simulink model "truesystem"  (R2020a)
settings: Solver=VariableStepAuto  StartTime=0.0  StopTime=stoptimetotal  RelTol=1e-3
values from neighbouring files (symbols this model uses):
  battery = load('params/battery.mat').battery    [prognostics.m]    (also in workspace_1.mat = )
  IC = load('params/IC_HoverAt10ftOcto.mat').IC    [prognostics.m]    (also in workspace_1.mat = )
  Motor1 = load('params/Motors/Motor1.mat').Motor    [prognostics.m]    (also in workspace_1.mat = )
  Motor2 = load('params/Motors/Motor2.mat').Motor    [prognostics.m]    (also in workspace_1.mat = )
  Motor3 = load('params/Motors/Motor3.mat').Motor    [prognostics.m]    (also in workspace_1.mat = )
  Motor4 = load('params/Motors/Motor4.mat').Motor    [prognostics.m]    (also in workspace_1.mat = )
  Motor5 = load('params/Motors/Motor5.mat').Motor    [prognostics.m]    (also in workspace_1.mat = )
  Motor6 = load('params/Motors/Motor6.mat').Motor    [prognostics.m]    (also in workspace_1.mat = )
  Motor7 = load('params/Motors/Motor7.mat').Motor    [prognostics.m]    (also in workspace_1.mat = )
  Motor8 = load('params/Motors/Motor8.mat').Motor    [prognostics.m]    (also in workspace_1.mat = )
  octomodel = load('params/octoModel.mat').octomodel    [prognostics.m]    (also in workspace_1.mat = )
  sampletimetraj = 1    [prognostics.m]    (also in workspace_1.mat)
undefined symbols (not defined in the file or in its folder): DiscIntNeverNeededParam, mu_wind
libraries: dspstat3 x9, sharedTrackingLibrary x4
(part 1 of 2)
settings Model: Creator=Researcher  LastModifiedBy=darrahts
settings DataIOCC: ReturnWorkspaceOutputs=off
settings DebuggingCC: ArithmeticOperatorsInVariantConditions=warning
settings SFSimCC: SimUseLocalCustomCode=off  CustomCodeUndefinedFunction=UseInterfaceOnly
settings RTWCC: RTWUseLocalCustomCode=off

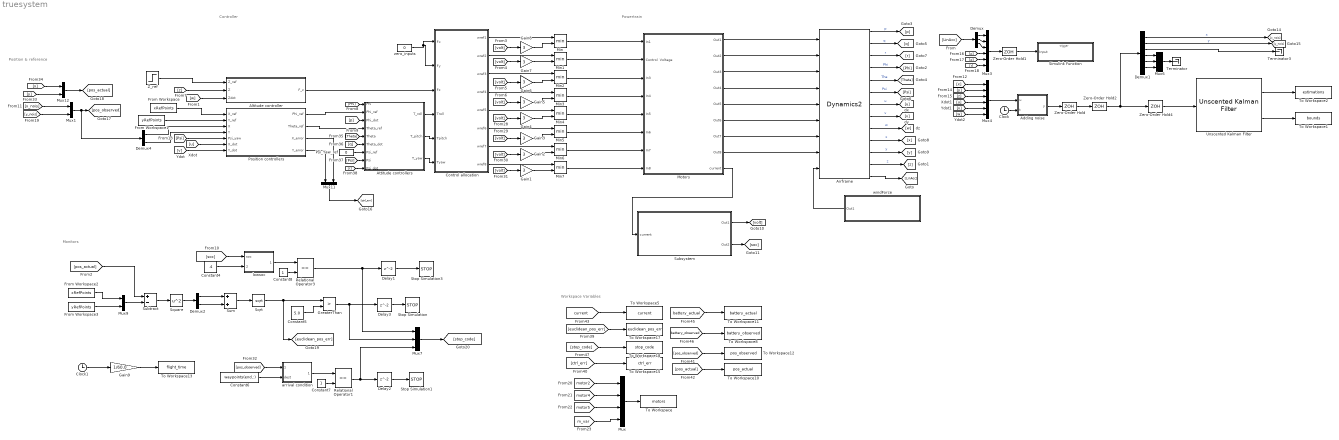
== system truesystem ==
  note: Powertrain
  note: Position & reference
  note: Controller
  note: Monitors
  note: Workspace Variables
  Adding noise : MATLAB Function  TreatAsAtomicUnit=on  SystemSampleTime=octomodel.sampletime
  Airframe : M-S-Function  FunctionName=Dynamics2  Parameters=octomodel, IC
  Altitude controller : Subsystem
  Attitude controllers : Subsystem
  Clock : Clock
  Clock1 : Clock
  Constant4 : Constant  Value=.4
  Constant5 : Constant  Value=5.0
  Constant6 : Constant  Value=waypoints(end,:)
  Constant7 : Constant
  Constant8 : Constant
  Control allocation : MATLAB Function  TreatAsAtomicUnit=on
  Delay1 : Delay
  Delay2 : Delay
  Delay3 : Delay
  Demux : Demux  Outputs=3
  Demux1 : Demux  Outputs=6
  Demux2 : Demux  Outputs=2
  Demux4 : Demux  Outputs=2
  From Workspace : FromWorkspace  VariableName=xRefPoints  SampleTime=sampletimetraj
  From Workspace1 : FromWorkspace  VariableName=yRefPoints  SampleTime=sampletimetraj
  From Workspace2 : FromWorkspace  VariableName=xRefPoints  SampleTime=sampletimetraj
  From Workspace3 : FromWorkspace  VariableName=yRefPoints  SampleTime=sampletimetraj
  Gain{1..8} (8 alike) : Gain  Gain=3
  Gain9 : Gain  Gain=1/60.0
  GreaterThan : RelationalOperator  Operator=>  OutDataTypeStr=boolean  RndMeth=Simplest
  Min{,1..7} (8 alike) : MinMax  Inputs=2
  Motors : Subsystem
  Mux : Mux
  Mux{1,9,11..12} (4 alike) : Mux  Inputs=2
  Mux3 : Mux  Inputs=6
  Mux4 : Mux  Inputs=6
  Mux6 : Mux  Inputs=3
  Mux7 : Mux  Inputs=3
  Position controllers : Subsystem
  Psi_Yaw_ref : Constant  Value=0
  Relational Operator1 : RelationalOperator  Operator===  OutDataTypeStr=boolean  RndMeth=Simplest
  Relational Operator3 : RelationalOperator  Operator===  OutDataTypeStr=boolean  RndMeth=Simplest
  Simulink Function : Subsystem  TreatAsAtomicUnit=on
  Sqrt : Sqrt  SaturateOnIntegerOverflow=on
  Square : Math  Operator=square  SaturateOnIntegerOverflow=on
  Stop Simulation : Stop
  Stop Simulation1 : Stop
  Stop Simulation3 : Stop
  Subsystem : Subsystem
  Subtract : Sum  Inputs=+-
  Sum : Sum
  Terminator : Terminator
  Terminator3 : Terminator
  To Workspace : ToWorkspace  VariableName=motors  SaveFormat=Timeseries  SampleTime=-1
  To Workspace1 : ToWorkspace  VariableName=bounds  SaveFormat=Timeseries  SampleTime=battery.dt
  To Workspace10 : ToWorkspace  VariableName=pos_actual  SaveFormat=Timeseries  SampleTime=-1
  To Workspace11 : ToWorkspace  VariableName=battery_actual  SaveFormat=Timeseries  SampleTime=-1
  To Workspace12 : ToWorkspace  VariableName=pos_observed  SaveFormat=Timeseries  SampleTime=-1
  To Workspace13 : ToWorkspace  VariableName=flight_time  SaveFormat=Timeseries  SampleTime=-1
  To Workspace15 : ToWorkspace  VariableName=ctrl_err  SaveFormat=Timeseries  SampleTime=-1
  To Workspace17 : ToWorkspace  VariableName=euclidean_pos_err  SaveFormat=Timeseries  SampleTime=-1
  To Workspace18 : ToWorkspace  VariableName=stop_code  SaveFormat=Timeseries  SampleTime=-1
  To Workspace2 : ToWorkspace  VariableName=estimations  SaveFormat=Timeseries  SampleTime=battery.dt
  To Workspace5 : ToWorkspace  VariableName=current  SaveFormat=Timeseries  SampleTime=-1
      settings: Save2DSignal=2-D array (concatenate along first dimension)
  To Workspace8 : ToWorkspace  VariableName=battery_observed  SaveFormat=Timeseries  SampleTime=-1
  Unscented Kalman Filter : sharedTrackingLibrary/Unscented Kalman Filter  StateTransitionFcn=stateTransitionFn  HasAdditiveProcessNoise=Additive  ProcessNoise=PositionEstimator.SigmaW  HasTimeVaryingProcessNoise=off  HasStateTransitionFcnExtraArgument=0  InitialState=IC.state  InitialStateCovariance=PositionEstimator.SigmaX  Alpha=0.75  Beta=2  Kappa=0  MeasurementFcn1=positionMeasTransitionFunction  HasMeasurementEnablePort1=off  HasAdditiveMeasurementNoise1=Additive  MeasurementNoise1=PositionEstimator.SigmaV  HasTimeVaryingMeasurementNoise1=off  HasMeasurementFcnExtraArgument1=0  MeasurementFcn2=myMeasurementFcn  HasMeasurementEnablePort2=off  HasAdditiveMeasurementNoise2=Additive  MeasurementNoise2=1  HasTimeVaryingMeasurementNoise2=off  HasMeasurementFcnExtraArgument2=0  MeasurementFcn3=myMeasurementFcn  HasMeasurementEnablePort3=off  HasAdditiveMeasurementNoise3=Additive  MeasurementNoise3=1  HasTimeVaryingMeasurementNoise3=off  HasMeasurementFcnExtraArgument3=0  MeasurementFcn4=myMeasurementFcn  HasMeasurementEnablePort4=off  HasAdditiveMeasurementNoise4=Additive  MeasurementNoise4=1  HasTimeVaryingMeasurementNoise4=off  HasMeasurementFcnExtraArgument4=0  MeasurementFcn5=myMeasurementFcn  HasMeasurementEnablePort5=off  HasAdditiveMeasurementNoise5=Additive  MeasurementNoise5=1  HasTimeVaryingMeasurementNoise5=off  HasMeasurementFcnExtraArgument5=0  EnableMultirate=off  StateTransitionFcnSampleTime=0.01  MeasurementFcn1SampleTime=1  MeasurementFcn2SampleTime=1  MeasurementFcn3SampleTime=1  MeasurementFcn4SampleTime=1  MeasurementFcn5SampleTime=1  UseCurrentEstimator=on  OutputStateCovariance=on  DataType=double  SampleTime=battery.dt  NumberOfMeasurements=1
      settings: SourceProductBaseCode=CT,DR,TF,ID,NV,AR,RO,VE
  Z_ref : Step  Before=3  After=3  SampleTime=0
  Zero-Order Hold : ZeroOrderHold
  Zero-Order Hold1 : ZeroOrderHold  SampleTime=octomodel.sampletime
  Zero-Order Hold2 : ZeroOrderHold  SampleTime=octomodel.sampletime
  Zero-Order Hold4 : ZeroOrderHold  SampleTime=battery.dt
  arrival condition : MATLAB Function  TreatAsAtomicUnit=on
  lowsoc : MATLAB Function  TreatAsAtomicUnit=on
  windForce : Subsystem
  zero_inputs : Constant  Value=0
  wires:
  Airframe/1 -> [p]  "p"
  Airframe/2 -> [q]  "q"
  Airframe/3 -> [r]  "r"
  Airframe/4 -> [Phi]  "Phi"
  Airframe/5 -> [Theta]  "The"
  Airframe/6 -> [Psi]  "Psi"
  Airframe/11 -> [y]  "y"
  Airframe/12 -> [z]  "z"
  Airframe/7 -> [u]  "u"
  Airframe/10 -> [x]  "x"
  Airframe/9 -> [w]  "w"
  Airframe/8 -> [v]  "v"
  Motors/3(Out3) -> Airframe/3
  Motors/1(Out1) -> Airframe/1
  Motors/8(Out8) -> Airframe/8
  Motors/7(Out7) -> Airframe/7
  Motors/6(Out6) -> Airframe/6
  Motors/5(Out5) -> Airframe/5
  Motors/4(Out4) -> Airframe/4
  Motors/2(Out2) -> Airframe/2
  Airframe/13 -> [LinAcc]
  [LinAcc] -> Demux/1
  Demux/1 -> Mux3/1
  Demux/2 -> Mux3/2
  Demux/3 -> Mux3/3
  [p] -> Mux3/4
  [q] -> Mux3/5
  [r] -> Mux3/6
  Zero-Order Hold1/1 -> Simulink Function/1(Input)
  Mux3/1 -> Zero-Order Hold1/1
  Clock/1 -> Adding noise/2(t)
  [y] -> Mux4/2
  Zero-Order Hold2/1 -> Zero-Order Hold4/1, Demux1/1
  Adding noise/1(y) -> Zero-Order Hold/1
  Unscented Kalman Filter/1 -> To Workspace2/1
  [x] -> Mux4/1
  [w] -> Mux4/6
  [z] -> Mux4/3
  [v] -> Mux4/5
  [u] -> Mux4/4
  Mux4/1 -> Adding noise/1(u)
  Unscented Kalman Filter/2 -> To Workspace1/1
  Zero-Order Hold/1 -> Zero-Order Hold2/1
  Demux1/3 -> Terminator3/1
  Mux6/1 -> Terminator/1
  Demux1/5 -> Mux6/2
  Demux1/4 -> Mux6/1
  Demux1/6 -> Mux6/3
  Demux1/2 -> [y_nois]  "y"
  Demux1/1 -> [x_nois]  "x"
  Zero-Order Hold4/1 -> Unscented Kalman Filter/1
  Control allocation/6(wref6) -> Min5/1
  [volt] -> Gain8/1
  Gain4/1 -> Min4/2
  Attitude controllers/1(T_roll) -> Control allocation/4(Troll)
  Min3/1 -> Motors/4(In4)
  Position controllers/1(Phi_ref) -> Attitude controllers/2(Phi_ref)
  [r] -> Attitude controllers/9(Psi_dot)
  Z_ref/1 -> Altitude controller/1(Z_ref)
  Gain5/1 -> Min3/2
  Gain1/1 -> Min7/2
  Attitude controllers/3(T_yaw) -> Control allocation/6(Tyaw)
  Control allocation/8(wref8) -> Min7/1
  Mux11/1 -> [ctrl_err]
  [x] -> Mux12/1
  Min7/1 -> Motors/8(In8)
  [Psi] -> Position controllers/5(Psi_yaw)
  [w] -> Altitude controller/3(Zdot)
  [u] -> Position controllers/6(X_dot)
  Demux4/1 -> Position controllers/3(X)
  From Workspace/1 -> Position controllers/1(X_ref)
  Control allocation/7(wref7) -> Min6/1
  Demux4/2 -> Position controllers/4(Y)
  Position controllers/3(X_error) -> Mux11/2
  Min2/1 -> Motors/3(In3)
  Control allocation/3(wref3) -> Min2/1
  [volt] -> Gain2/1
  Min4/1 -> Motors/5(In5)
  Attitude controllers/2(T_pitch) -> Control allocation/5(Tpitch)
  [Theta] -> Attitude controllers/5(Theta)
  Position controllers/2(Theta_ref) -> Attitude controllers/4(Theta_ref)
  Control allocation/1(wref1) -> Min/1
  Altitude controller/1(F_z) -> Control allocation/3(Fz)
  [y] -> Mux12/2
  [Phi] -> Attitude controllers/1(Phi)
  [z] -> Altitude controller/2(Z)
  [volt] -> Gain5/1
  Position controllers/4(Y_error) -> Mux11/1
  Gain2/1 -> Min6/2
  Min5/1 -> Motors/6(In6)
  Control allocation/4(wref4) -> Min3/1
  Min1/1 -> Motors/2(Control  Voltage)
  [volt] -> Gain4/1
  Control allocation/5(wref5) -> Min4/1
  [volt] -> Gain3/1
  Control allocation/2(wref2) -> Min1/1
  From Workspace1/1 -> Position controllers/2(Y_ref)
  [v] -> Position controllers/7(Y_dot)
  [Psi] -> Attitude controllers/8(Psi)
  [volt] -> Gain1/1
  Min6/1 -> Motors/7(In7)
  [volt] -> Gain7/1
  zero_inputs/1 -> Control allocation/1(Fx), Control allocation/2(Fy)
  Min/1 -> Motors/1(In1)
  Gain8/1 -> Min/2
  [q] -> Attitude controllers/6(Theta_dot)
  Psi_Yaw_ref/1 -> Attitude controllers/7(Psi_ref)
  [p] -> Attitude controllers/3(Phi_dot)
  [volt] -> Gain6/1
  Gain3/1 -> Min5/2
  Gain7/1 -> Min1/2
  Mux12/1 -> [pos_actual]
  Gain6/1 -> Min2/2
  Constant7/1 -> Relational Operator1/2
  Mux7/1 -> [stop_code]
  lowsoc/1(lowsoc) -> Relational Operator3/1
  Constant6/1 -> arrival condition/2(dest)
  Demux2/2 -> Sum/2
  Delay2/1 -> Stop Simulation1/1
  Constant5/1 -> GreaterThan/2
  Gain9/1 -> To Workspace13/1
  arrival condition/1(arrived) -> Relational Operator1/1
  Demux2/1 -> Sum/1
  [pos_actual] -> Subtract/1
  Mux9/1 -> Subtract/2
  Delay1/1 -> Stop Simulation3/1
  From Workspace3/1 -> Mux9/2
  Constant4/1 -> lowsoc/2(threshold)
  Clock1/1 -> Gain9/1
  Sum/1 -> Sqrt/1
  [soc] -> lowsoc/1(soc)
  GreaterThan/1 -> Mux7/2, Delay3/1
  Sqrt/1 -> [euclidean_pos_err], GreaterThan/1
  Square/1 -> Demux2/1
  Subtract/1 -> Square/1
  From Workspace2/1 -> Mux9/1
  Constant8/1 -> Relational Operator3/2
  [pos_observed] -> arrival condition/1(currentpos)
  Relational Operator1/1 -> Mux7/3, Delay2/1
  Delay3/1 -> Stop Simulation/1
  Relational Operator3/1 -> Mux7/1, Delay1/1
  [stop_code] -> To Workspace18/1
  [pos_actual] -> To Workspace10/1
  [pos_observed] -> To Workspace12/1
  [ctrl_err] -> To Workspace15/1
  [battery_actual] -> To Workspace11/1
  [current] -> To Workspace5/1
  [battery_observed] -> To Workspace8/1
  [euclidean_pos_err] -> To Workspace17/1
  Motors/9(current) -> Subsystem/1(current)
  Subsystem/1(Out1) -> [volt]
  Subsystem/2(Out2) -> [soc]
  Mux1/1 -> Demux4/1, [pos_observed]
  [x_nois] -> Mux1/1
  [y_nois] -> Mux1/2
  windForce/1(Out1) -> Airframe/9
  [motor2] -> Mux/1
  [m_var] -> Mux/4
  [motor5] -> Mux/3
  [motor4] -> Mux/2
  Mux/1 -> To Workspace/1

== system truesystem/Altitude controller ==
  Z_ref : Inport
  Z : Inport  Port=2
  Zdot : Inport  Port=3
  Add : Sum  Inputs=+++
  Add2 : Sum  Inputs=+-
  Constant2 : Constant  Value=octomodel.g*octomodel.mass
  Kdz : Gain  Gain=-3
  Kpz : Gain  Gain=-10
  mass : Gain  Gain=octomodel.mass
  mass1 : Gain  Gain=octomodel.mass
  F_z : Outport  VectorParamsAs1DForOutWhenUnconnected=off
  wires:
  Add2/1 -> Kpz/1
  Constant2/1 -> Add/1
  Z/1 -> Add2/1
  Add/1 -> F_z/1
  Z_ref/1 -> Add2/2
  Zdot/1 -> Kdz/1
  Kpz/1 -> mass/1
  Kdz/1 -> mass1/1
  mass1/1 -> Add/3
  mass/1 -> Add/2

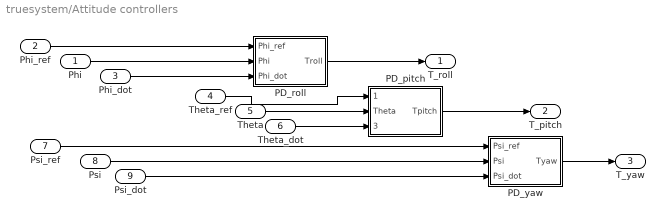
== system truesystem/Attitude controllers ==
  Phi : Inport
  Phi_ref : Inport  Port=2
  Phi_dot : Inport  Port=3
  Theta_ref : Inport  Port=4
  Theta : Inport  Port=5
  Theta_dot : Inport  Port=6
  Psi_ref : Inport  Port=7
  Psi : Inport  Port=8
  Psi_dot : Inport  Port=9
  PD_pitch : Subsystem
  PD_roll : Subsystem
  PD_yaw : Subsystem
  T_roll : Outport  VectorParamsAs1DForOutWhenUnconnected=off
  T_pitch : Outport  Port=2  VectorParamsAs1DForOutWhenUnconnected=off
  T_yaw : Outport  Port=3  VectorParamsAs1DForOutWhenUnconnected=off
  wires:
  PD_yaw/1(Tyaw) -> T_yaw/1
  PD_roll/1(Troll) -> T_roll/1
  Theta_ref/1 -> PD_pitch/1(Theta_ref)
  Theta_dot/1 -> PD_pitch/3(Theta_dot)
  PD_pitch/1(Tpitch) -> T_pitch/1
  Phi/1 -> PD_roll/2(Phi)
  Psi_dot/1 -> PD_yaw/3(Psi_dot)
  Psi_ref/1 -> PD_yaw/1(Psi_ref)
  Theta/1 -> PD_pitch/2(Theta)
  Phi_dot/1 -> PD_roll/3(Phi_dot)
  Psi/1 -> PD_yaw/2(Psi)
  Phi_ref/1 -> PD_roll/1(Phi_ref)

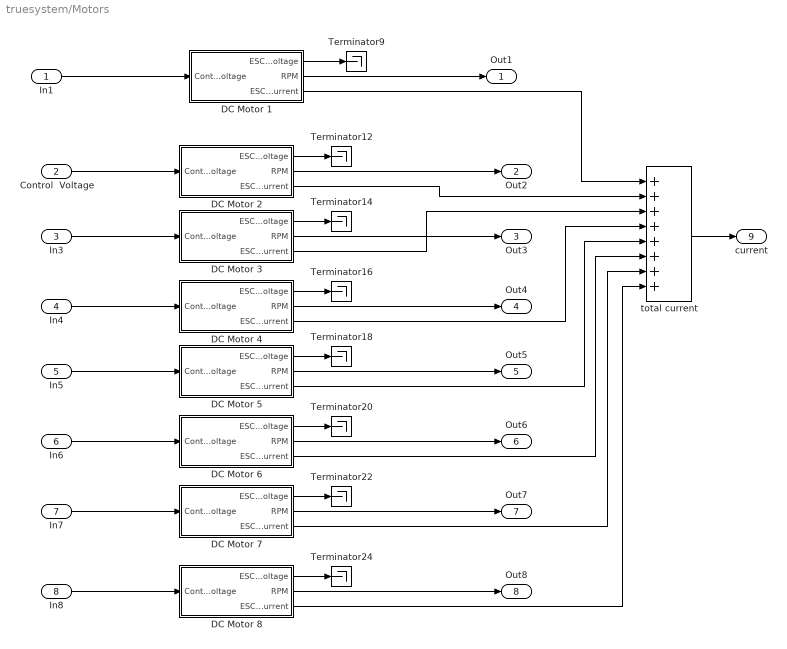
== system truesystem/Motors ==
  In1 : Inport
  Control  Voltage : Inport  Port=2
  In3 : Inport  Port=3
  In4 : Inport  Port=4
  In5 : Inport  Port=5
  In6 : Inport  Port=6
  In7 : Inport  Port=7
  In8 : Inport  Port=8
  "DC Motor 1 " : Subsystem
  DC Motor 2 : Subsystem
  DC Motor 3 : Subsystem
  DC Motor 4 : Subsystem
  DC Motor 5 : Subsystem
  DC Motor 6 : Subsystem
  DC Motor 7 : Subsystem
  DC Motor 8 : Subsystem
  Terminator{9,12,14,16,18,20,22,24} (8 alike) : Terminator
  total current : Sum  Inputs=++++++++
  Out1 : Outport  VectorParamsAs1DForOutWhenUnconnected=off
  Out2 : Outport  Port=2  VectorParamsAs1DForOutWhenUnconnected=off
  Out3 : Outport  Port=3  VectorParamsAs1DForOutWhenUnconnected=off
  Out4 : Outport  Port=4  VectorParamsAs1DForOutWhenUnconnected=off
  Out5 : Outport  Port=5  VectorParamsAs1DForOutWhenUnconnected=off
  Out6 : Outport  Port=6  VectorParamsAs1DForOutWhenUnconnected=off
  Out7 : Outport  Port=7  VectorParamsAs1DForOutWhenUnconnected=off
  Out8 : Outport  Port=8  VectorParamsAs1DForOutWhenUnconnected=off
  current : Outport  Port=9  VectorParamsAs1DForOutWhenUnconnected=off
  wires:
  DC Motor 5/1(ESC Voltage) -> Terminator18/1
  DC Motor 6/3(ESC Current) -> total current/6
  DC Motor 7/3(ESC Current) -> total current/7
  DC Motor 7/1(ESC Voltage) -> Terminator22/1
  DC Motor 6/1(ESC Voltage) -> Terminator20/1
  DC Motor 5/3(ESC Current) -> total current/5
  DC Motor 8/3(ESC Current) -> total current/8
  "DC Motor 1 "/3(ESC Current) -> total current/1
  "DC Motor 1 "/1(ESC Voltage) -> Terminator9/1
  DC Motor 2/3(ESC Current) -> total current/2
  DC Motor 2/1(ESC Voltage) -> Terminator12/1
  DC Motor 3/1(ESC Voltage) -> Terminator14/1
  DC Motor 4/3(ESC Current) -> total current/4
  DC Motor 3/3(ESC Current) -> total current/3
  DC Motor 5/2(RPM) -> Out5/1
  DC Motor 4/1(ESC Voltage) -> Terminator16/1
  DC Motor 8/1(ESC Voltage) -> Terminator24/1
  DC Motor 7/2(RPM) -> Out7/1
  DC Motor 2/2(RPM) -> Out2/1
  DC Motor 3/2(RPM) -> Out3/1
  DC Motor 4/2(RPM) -> Out4/1
  DC Motor 6/2(RPM) -> Out6/1
  DC Motor 8/2(RPM) -> Out8/1
  "DC Motor 1 "/2(RPM) -> Out1/1
  In1/1 -> "DC Motor 1 "/1(Control  Voltage)
  In7/1 -> DC Motor 7/1(Control  Voltage)
  In8/1 -> DC Motor 8/1(Control  Voltage)
  In6/1 -> DC Motor 6/1(Control  Voltage)
  In5/1 -> DC Motor 5/1(Control  Voltage)
  In4/1 -> DC Motor 4/1(Control  Voltage)
  In3/1 -> DC Motor 3/1(Control  Voltage)
  Control  Voltage/1 -> DC Motor 2/1(Control  Voltage)
  total current/1 -> current/1

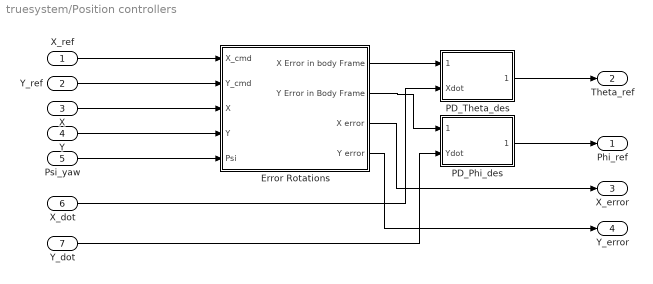
== system truesystem/Position controllers ==
  X_ref : Inport
  Y_ref : Inport  Port=2
  X : Inport  Port=3
  Y : Inport  Port=4
  Psi_yaw : Inport  Port=5
  X_dot : Inport  Port=6
  Y_dot : Inport  Port=7
  Error Rotations : Subsystem
  PD_Phi_des : Subsystem
  PD_Theta_des : Subsystem
  Phi_ref : Outport  VectorParamsAs1DForOutWhenUnconnected=off
  Theta_ref : Outport  Port=2  VectorParamsAs1DForOutWhenUnconnected=off
  X_error : Outport  Port=3  VectorParamsAs1DForOutWhenUnconnected=off
  Y_error : Outport  Port=4  VectorParamsAs1DForOutWhenUnconnected=off
  wires:
  Y/1 -> Error Rotations/4(Y)
  Y_ref/1 -> Error Rotations/2(Y_cmd)
  Error Rotations/4("Y error ") -> Y_error/1
  Error Rotations/3(X error) -> X_error/1
  Error Rotations/1(X Error in body Frame) -> PD_Theta_des/1(Xdot_ref)
  X/1 -> Error Rotations/3(X)
  Y_dot/1 -> PD_Phi_des/2(Ydot)
  PD_Phi_des/1(Phi_des) -> Phi_ref/1
  Error Rotations/2(Y Error in Body Frame) -> PD_Phi_des/1(Ydot_ref)
  Psi_yaw/1 -> Error Rotations/5(Psi)
  PD_Theta_des/1(Theta_des) -> Theta_ref/1
  X_dot/1 -> PD_Theta_des/2(Xdot)
  X_ref/1 -> Error Rotations/1(X_cmd)

== system truesystem/Simulink Function ==
  Input : Inport  PortDimensions=6
  stateTransitionFn : TriggerPort  TriggerType=function-call  IsSimulinkFunction=on  FunctionName=stateTransitionFn  VariantControl=(inherit)
  MATLAB Function : MATLAB Function  TreatAsAtomicUnit=on
  x : ArgIn  DisableCoverage=on  PortDimensions=9  ArgumentName=x
  xNext : ArgOut  DisableCoverage=on  PortDimensions=9  ArgumentName=xNext
  wires:
  x/1 -> MATLAB Function/1("x ")
  MATLAB Function/1(x) -> xNext/1
  Input/1 -> MATLAB Function/2(u)

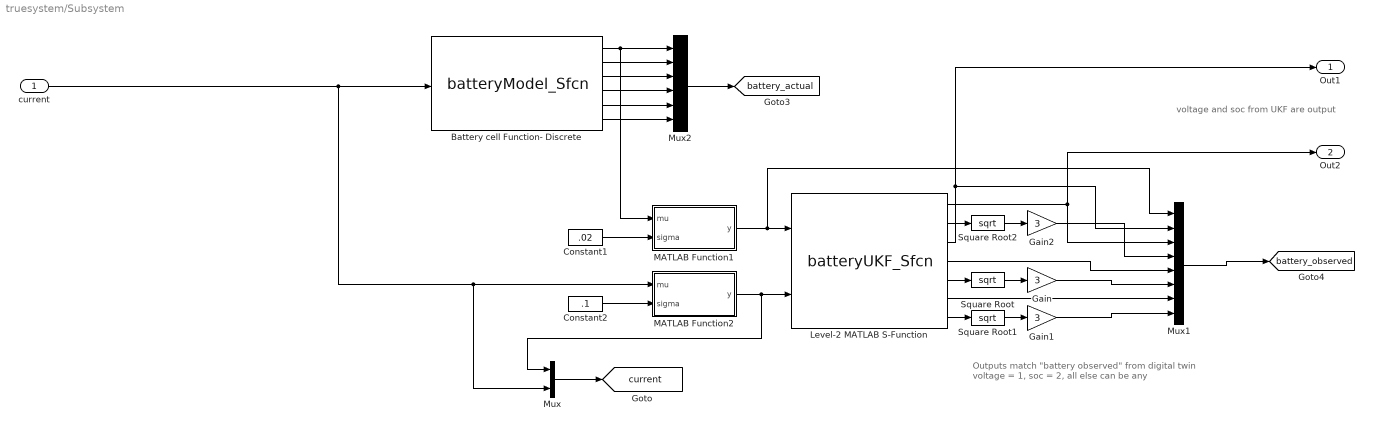
== system truesystem/Subsystem ==
  note: voltage and soc from UKF are output
  note: Outputs match "battery observed" from digital twin
      | voltage = 1, soc = 2, all else can be any
  current : Inport
  Battery cell Function- Discrete : M-S-Function  FunctionName=batteryModel_Sfcn  Parameters=battery, battery.dt
      mask Display:
      | port_label('input', 1, 'current');
      | port_label('output', 1, 'voltage');
      | port_label('output', 2, 'soc');
      | port_label('output', 3, 'R0');
      | port_label('output', 4, 'Ir');
      | port_label('output', 5, 'h');
      | port_label('output', 6, 'Q');
      | 
      | disp("Battery Cell");
  Constant1 : Constant  Value=.02
  Constant2 : Constant  Value=.1
  Gain : Gain  Gain=3
  Gain1 : Gain  Gain=3
  Gain2 : Gain  Gain=3
  Level-2 MATLAB S-Function : M-S-Function  FunctionName=batteryUKF_Sfcn  Parameters=battery, battery.dt, ukfBatteryParams
      mask Display:
      | port_label('input', 1, 'voltage');
      | port_label('input', 2, 'current');
      | port_label('output', 1, 'soc_hat');
      | port_label('output', 2, 'soc_bound');
      | port_label('output', 3, 'voltage_hat');
      | port_label('output', 4, 'r0_hat');
      | port_label('output', 5, 'r0_bound');
      | port_label('output', 6, 'q_hat');
      | port_label('output', 7, 'q_bound');
      | 
      | disp("UKF");
  MATLAB Function1 : MATLAB Function  TreatAsAtomicUnit=on
  MATLAB Function2 : MATLAB Function  TreatAsAtomicUnit=on
  Mux : Mux  Inputs=2
  Mux1 : Mux  Inputs=8
  Mux2 : Mux  Inputs=6
  Square Root : Sqrt  SaturateOnIntegerOverflow=on
  Square Root1 : Sqrt  SaturateOnIntegerOverflow=on
  Square Root2 : Sqrt  SaturateOnIntegerOverflow=on
  Out1 : Outport
  Out2 : Outport  Port=2
  tag scope: battery_actual=global, battery_observed=global, current=global
  wires:
  MATLAB Function1/1(y) -> Mux1/1, Level-2 MATLAB S-Function/1
  Constant1/1 -> MATLAB Function1/2(sigma)
  Level-2 MATLAB S-Function/5 -> Square Root/1
  Square Root/1 -> Gain/1
  Battery cell Function- Discrete/6 -> Mux2/6
  Battery cell Function- Discrete/1 -> MATLAB Function1/1(mu), Mux2/1
  Battery cell Function- Discrete/5 -> Mux2/5
  Battery cell Function- Discrete/2 -> Mux2/2
  Battery cell Function- Discrete/4 -> Mux2/4
  Mux2/1 -> [battery_actual]
  Battery cell Function- Discrete/3 -> Mux2/3
  Square Root1/1 -> Gain1/1
  Square Root2/1 -> Gain2/1
  Level-2 MATLAB S-Function/2 -> Square Root2/1
  Level-2 MATLAB S-Function/7 -> Square Root1/1
  Level-2 MATLAB S-Function/3 -> Mux1/2, Out1/1
  Level-2 MATLAB S-Function/1 -> Out2/1, Mux1/3
  Gain2/1 -> Mux1/4
  Level-2 MATLAB S-Function/4 -> Mux1/5
  Gain/1 -> Mux1/6
  Level-2 MATLAB S-Function/6 -> Mux1/7
  Gain1/1 -> Mux1/8
  Mux1/1 -> [battery_observed]
  Constant2/1 -> MATLAB Function2/2(sigma)
  current/1 -> Mux/2, MATLAB Function2/1(mu), Battery cell Function- Discrete/1
  MATLAB Function2/1(y) -> Mux/1, Level-2 MATLAB S-Function/2
  Mux/1 -> [current]

== system truesystem/windForce ==
  Constant10 : Constant  Value=[0;0;0]
  Gain : Gain  Gain=.5
  Manual Switch1 : ManualSwitch  CurrentSetting=0
  Mux9 : Mux  Inputs=3
  Random Number : RandomNumber  Mean=mu_wind  Variance=.5  Seed=37
  Random Number1 : RandomNumber  Mean=mu_wind  Variance=.5  Seed=41
  Random Number2 : RandomNumber  Mean=mu_wind  Variance=.5
  Out1 : Outport
  wires:
  Random Number1/1 -> Mux9/2
  Mux9/1 -> Gain/1
  Manual Switch1/1 -> Out1/1
  Random Number2/1 -> Mux9/3
  Random Number/1 -> Mux9/1
  Constant10/1 -> Manual Switch1/1
  Gain/1 -> Manual Switch1/2

== system truesystem/Attitude controllers/PD_pitch ==
  Theta_ref : Inport
  Theta : Inport  Port=2
  Theta_dot : Inport  Port=3
  Add : Sum  Inputs=-+
  Gain : Gain  Gain=3
  Gain1 : Gain
  Gain2 : Gain  Gain=-1
  Sum : Sum  Inputs=|++
  Tpitch : Outport  VectorParamsAs1DForOutWhenUnconnected=off
  wires:
  Gain2/1 -> Tpitch/1
  Gain/1 -> Sum/1
  Theta/1 -> Add/2
  Add/1 -> Gain/1
  Gain1/1 -> Sum/2
  Sum/1 -> Gain2/1
  Theta_dot/1 -> Gain1/1
  Theta_ref/1 -> Add/1

== system truesystem/Attitude controllers/PD_roll ==
  Phi_ref : Inport
  Phi : Inport  Port=2
  Phi_dot : Inport  Port=3
  Add : Sum  Inputs=-+
  Gain : Gain  Gain=3
  Gain1 : Gain
  Gain2 : Gain  Gain=-1
  Sum : Sum  Inputs=|++
  Troll : Outport  VectorParamsAs1DForOutWhenUnconnected=off
  wires:
  Phi_ref/1 -> Add/1
  Phi_dot/1 -> Gain1/1
  Sum/1 -> Gain2/1
  Gain1/1 -> Sum/2
  Add/1 -> Gain/1
  Phi/1 -> Add/2
  Gain/1 -> Sum/1
  Gain2/1 -> Troll/1

== system truesystem/Attitude controllers/PD_yaw ==
  Psi_ref : Inport
  Psi : Inport  Port=2
  Psi_dot : Inport  Port=3
  Add : Sum  Inputs=-+
  Gain : Gain  Gain=3
  Gain1 : Gain
  Gain2 : Gain  Gain=-1
  Sum : Sum  Inputs=|++
  Tyaw : Outport  VectorParamsAs1DForOutWhenUnconnected=off
  wires:
  Psi_ref/1 -> Add/1
  Psi_dot/1 -> Gain1/1
  Sum/1 -> Gain2/1
  Gain1/1 -> Sum/2
  Add/1 -> Gain/1
  Psi/1 -> Add/2
  Gain/1 -> Sum/1
  Gain2/1 -> Tyaw/1

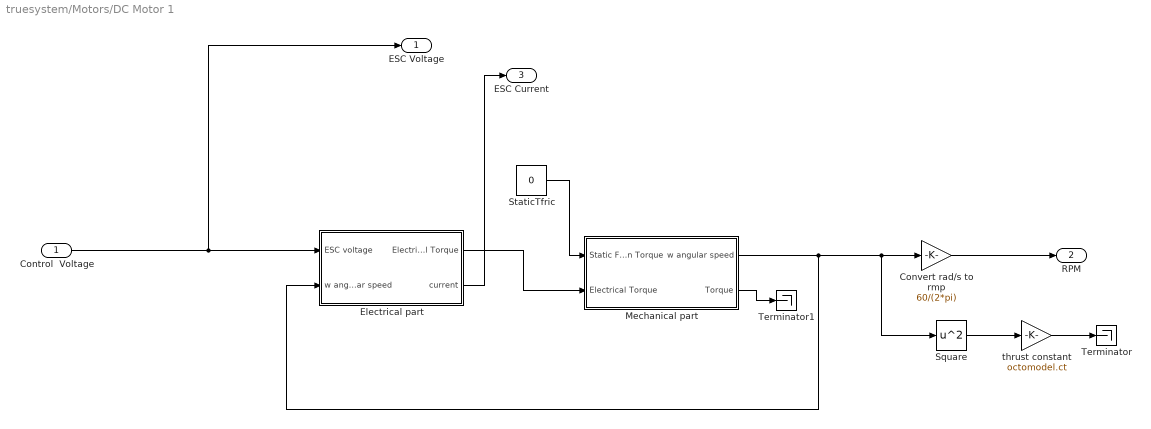
== system truesystem/Motors/DC Motor 1  ==
  Control  Voltage : Inport
  Convert rad/s to rmp : Gain  Gain=60/(2*pi)
  Electrical part : Subsystem
  Mechanical part : Subsystem
  Square : Math  Operator=square  SaturateOnIntegerOverflow=on
  StaticTfric : Constant  Value=0
  Terminator : Terminator
  Terminator1 : Terminator
  thrust constant : Gain  Gain=octomodel.ct
  ESC Voltage : Outport  VectorParamsAs1DForOutWhenUnconnected=off
  RPM : Outport  Port=2  VectorParamsAs1DForOutWhenUnconnected=off
  ESC Current : Outport  Port=3  VectorParamsAs1DForOutWhenUnconnected=off
  wires:
  Electrical part/1(Electrical Torque) -> Mechanical part/2(Electrical Torque)
  StaticTfric/1 -> Mechanical part/1(Static Friction Torque)
  Convert rad/s to rmp/1 -> RPM/1
  Square/1 -> thrust constant/1
  thrust constant/1 -> Terminator/1
  Mechanical part/2(Torque) -> Terminator1/1
  Electrical part/2(current) -> ESC Current/1
  Control  Voltage/1 -> ESC Voltage/1, Electrical part/1(ESC voltage)
  Mechanical part/1(w angular speed) -> Electrical part/2(w angular speed), Square/1, Convert rad/s to rmp/1

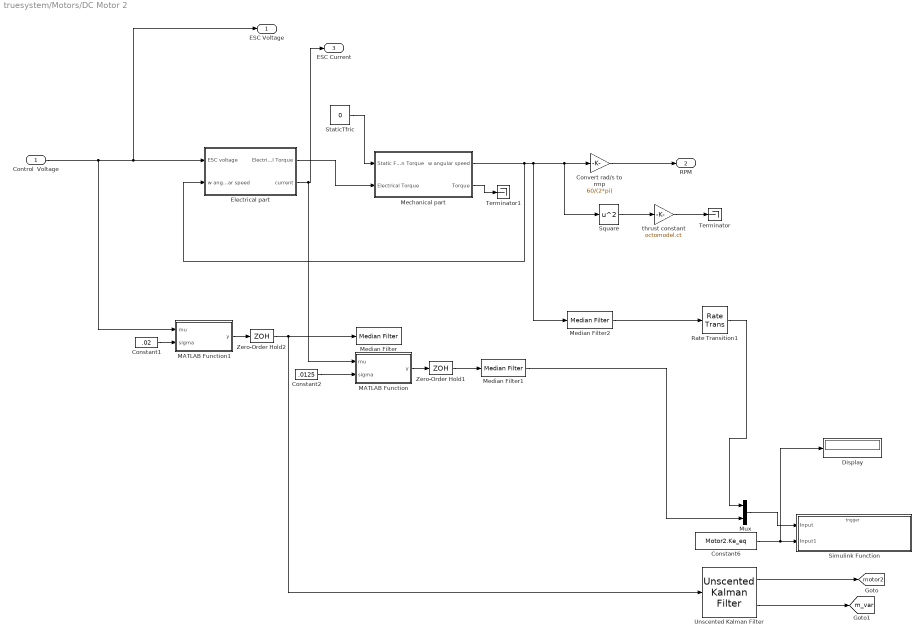
== system truesystem/Motors/DC Motor 2 ==
  Control  Voltage : Inport
  Constant1 : Constant  Value=.02
  Constant2 : Constant  Value=.0125
  Constant6 : Constant  Value=Motor2.Ke_eq
  Convert rad/s to rmp : Gain  Gain=60/(2*pi)
  Display : Display
  Electrical part : Subsystem
  MATLAB Function : MATLAB Function  TreatAsAtomicUnit=on
  MATLAB Function1 : MATLAB Function  TreatAsAtomicUnit=on
  Mechanical part : Subsystem
  Median Filter : dspstat3/Median Filter  WindowLength=5  SimulateUsing=Interpreted execution
      settings: SourceProductBaseCode=DS
  Median Filter1 : dspstat3/Median Filter  WindowLength=5  SimulateUsing=Interpreted execution
      settings: SourceProductBaseCode=DS
  Median Filter2 : dspstat3/Median Filter  WindowLength=5  SimulateUsing=Interpreted execution
      settings: SourceProductBaseCode=DS
  Mux : Mux  Inputs=2
  Rate Transition1 : RateTransition  OutPortSampleTime=octomodel.sampletime
  Simulink Function : Subsystem  TreatAsAtomicUnit=on
  Square : Math  Operator=square  SaturateOnIntegerOverflow=on
  StaticTfric : Constant  Value=0
  Terminator : Terminator
  Terminator1 : Terminator
  Unscented Kalman Filter : sharedTrackingLibrary/Unscented Kalman Filter  StateTransitionFcn=MotorTransitionFcn  HasAdditiveProcessNoise=Additive  ProcessNoise=0.001  HasTimeVaryingProcessNoise=off  HasStateTransitionFcnExtraArgument=0  InitialState=MotorEstimator.Rinit  InitialStateCovariance=0.001  Alpha=0.0001  Beta=2  Kappa=0  MeasurementFcn1=MotorMeasurementFcn2  HasMeasurementEnablePort1=off  HasAdditiveMeasurementNoise1=Additive  MeasurementNoise1=0.02  HasTimeVaryingMeasurementNoise1=off  HasMeasurementFcnExtraArgument1=0  MeasurementFcn2=myMeasurementFcn  HasMeasurementEnablePort2=off  HasAdditiveMeasurementNoise2=Additive  MeasurementNoise2=1  HasTimeVaryingMeasurementNoise2=off  HasMeasurementFcnExtraArgument2=0  MeasurementFcn3=myMeasurementFcn  HasMeasurementEnablePort3=off  HasAdditiveMeasurementNoise3=Additive  MeasurementNoise3=1  HasTimeVaryingMeasurementNoise3=off  HasMeasurementFcnExtraArgument3=0  MeasurementFcn4=myMeasurementFcn  HasMeasurementEnablePort4=off  HasAdditiveMeasurementNoise4=Additive  MeasurementNoise4=1  HasTimeVaryingMeasurementNoise4=off  HasMeasurementFcnExtraArgument4=0  MeasurementFcn5=myMeasurementFcn  HasMeasurementEnablePort5=off  HasAdditiveMeasurementNoise5=Additive  MeasurementNoise5=1  HasTimeVaryingMeasurementNoise5=off  HasMeasurementFcnExtraArgument5=0  EnableMultirate=off  StateTransitionFcnSampleTime=1  MeasurementFcn1SampleTime=1  MeasurementFcn2SampleTime=1  MeasurementFcn3SampleTime=1  MeasurementFcn4SampleTime=1  MeasurementFcn5SampleTime=1  UseCurrentEstimator=on  OutputStateCovariance=on  DataType=double  SampleTime=octomodel.sampletime  NumberOfMeasurements=1
      settings: SourceProductBaseCode=CT,DR,TF,ID,NV,AR,RO,VE
  Zero-Order Hold1 : ZeroOrderHold  SampleTime=octomodel.sampletime
  Zero-Order Hold2 : ZeroOrderHold  SampleTime=octomodel.sampletime
  thrust constant : Gain  Gain=octomodel.ct
  ESC Voltage : Outport  VectorParamsAs1DForOutWhenUnconnected=off
  RPM : Outport  Port=2  VectorParamsAs1DForOutWhenUnconnected=off
  ESC Current : Outport  Port=3  VectorParamsAs1DForOutWhenUnconnected=off
  tag scope: m_var=global, motor2=global
  wires:
  Square/1 -> thrust constant/1
  thrust constant/1 -> Terminator/1
  Convert rad/s to rmp/1 -> RPM/1
  StaticTfric/1 -> Mechanical part/1(Static Friction Torque)
  Electrical part/1(Electrical Torque) -> Mechanical part/2(Electrical Torque)
  Mechanical part/2(Torque) -> Terminator1/1
  Control  Voltage/1 -> MATLAB Function1/1(mu), Electrical part/1(ESC voltage), ESC Voltage/1
  Zero-Order Hold1/1 -> Median Filter1/1
  Mechanical part/1(w angular speed) -> Median Filter2/1, Convert rad/s to rmp/1, Square/1, Electrical part/2(w angular speed)
  Electrical part/2(current) -> MATLAB Function/1(mu), ESC Current/1
  MATLAB Function/1(y) -> Zero-Order Hold1/1
  Constant2/1 -> MATLAB Function/2(sigma)
  Constant1/1 -> MATLAB Function1/2(sigma)
  MATLAB Function1/1(y) -> Zero-Order Hold2/1
  Median Filter2/1 -> Rate Transition1/1
  Median Filter1/1 -> Mux/2
  Mux/1 -> Simulink Function/1(Input)
  Rate Transition1/1 -> Mux/1
  Unscented Kalman Filter/1 -> [motor2]
  Constant6/1 -> Display/1, Simulink Function/2(Input1)
  Zero-Order Hold2/1 -> Unscented Kalman Filter/1, Median Filter/1
  Unscented Kalman Filter/2 -> [m_var]

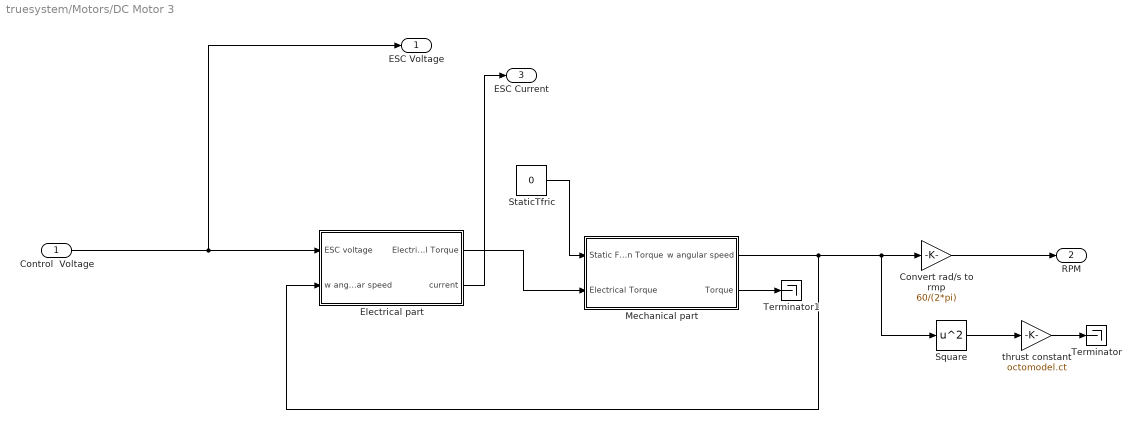
== system truesystem/Motors/DC Motor 3 ==
  Control  Voltage : Inport
  Convert rad/s to rmp : Gain  Gain=60/(2*pi)
  Electrical part : Subsystem
  Mechanical part : Subsystem
  Square : Math  Operator=square  SaturateOnIntegerOverflow=on
  StaticTfric : Constant  Value=0
  Terminator : Terminator
  Terminator1 : Terminator
  thrust constant : Gain  Gain=octomodel.ct
  ESC Voltage : Outport  VectorParamsAs1DForOutWhenUnconnected=off
  RPM : Outport  Port=2  VectorParamsAs1DForOutWhenUnconnected=off
  ESC Current : Outport  Port=3  VectorParamsAs1DForOutWhenUnconnected=off
  wires:
  Electrical part/1(Electrical Torque) -> Mechanical part/2(Electrical Torque)
  StaticTfric/1 -> Mechanical part/1(Static Friction Torque)
  Control  Voltage/1 -> ESC Voltage/1, Electrical part/1(ESC voltage)
  Electrical part/2(current) -> ESC Current/1
  Convert rad/s to rmp/1 -> RPM/1
  Mechanical part/1(w angular speed) -> Electrical part/2(w angular speed), Square/1, Convert rad/s to rmp/1
  thrust constant/1 -> Terminator/1
  Square/1 -> thrust constant/1
  Mechanical part/2(Torque) -> Terminator1/1

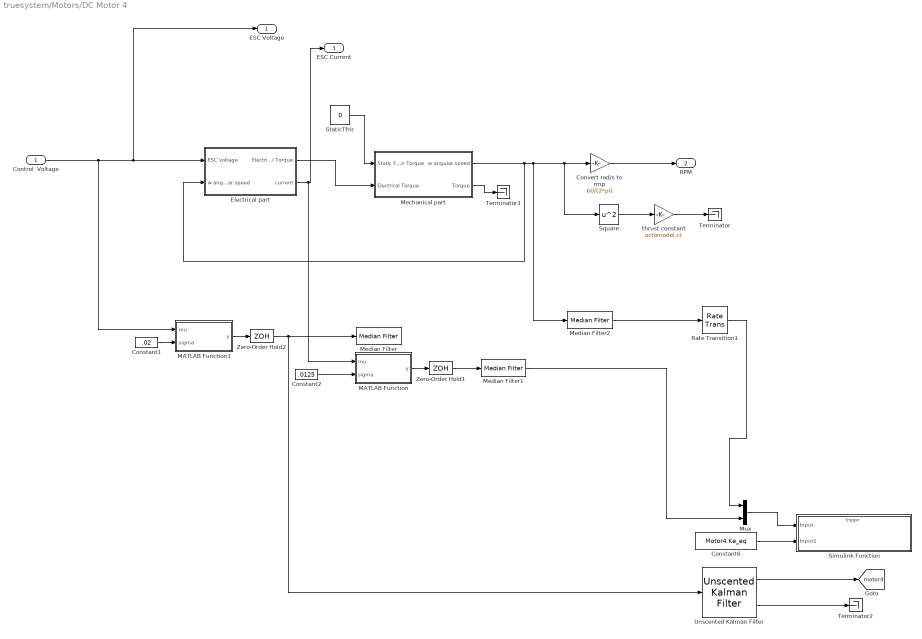
== system truesystem/Motors/DC Motor 4 ==
  Control  Voltage : Inport
  Constant1 : Constant  Value=.02
  Constant2 : Constant  Value=.0125
  Constant6 : Constant  Value=Motor4.Ke_eq
  Convert rad/s to rmp : Gain  Gain=60/(2*pi)
  Electrical part : Subsystem
  MATLAB Function : MATLAB Function  TreatAsAtomicUnit=on
  MATLAB Function1 : MATLAB Function  TreatAsAtomicUnit=on
  Mechanical part : Subsystem
  Median Filter : dspstat3/Median Filter  WindowLength=5  SimulateUsing=Interpreted execution
      settings: SourceProductBaseCode=DS
  Median Filter1 : dspstat3/Median Filter  WindowLength=5  SimulateUsing=Interpreted execution
      settings: SourceProductBaseCode=DS
  Median Filter2 : dspstat3/Median Filter  WindowLength=5  SimulateUsing=Interpreted execution
      settings: SourceProductBaseCode=DS
  Mux : Mux  Inputs=2
  Rate Transition1 : RateTransition  OutPortSampleTime=octomodel.sampletime
  Simulink Function : Subsystem  TreatAsAtomicUnit=on
  Square : Math  Operator=square  SaturateOnIntegerOverflow=on
  StaticTfric : Constant  Value=0
  Terminator : Terminator
  Terminator1 : Terminator
  Terminator2 : Terminator
  Unscented Kalman Filter : sharedTrackingLibrary/Unscented Kalman Filter  StateTransitionFcn=MotorTransitionFcn  HasAdditiveProcessNoise=Additive  ProcessNoise=0.001  HasTimeVaryingProcessNoise=off  HasStateTransitionFcnExtraArgument=0  InitialState=MotorEstimator.Rinit  InitialStateCovariance=0.001  Alpha=0.0001  Beta=2  Kappa=0  MeasurementFcn1=MotorMeasurementFcn4  HasMeasurementEnablePort1=off  HasAdditiveMeasurementNoise1=Additive  MeasurementNoise1=0.02  HasTimeVaryingMeasurementNoise1=off  HasMeasurementFcnExtraArgument1=0  MeasurementFcn2=myMeasurementFcn  HasMeasurementEnablePort2=off  HasAdditiveMeasurementNoise2=Additive  MeasurementNoise2=1  HasTimeVaryingMeasurementNoise2=off  HasMeasurementFcnExtraArgument2=0  MeasurementFcn3=myMeasurementFcn  HasMeasurementEnablePort3=off  HasAdditiveMeasurementNoise3=Additive  MeasurementNoise3=1  HasTimeVaryingMeasurementNoise3=off  HasMeasurementFcnExtraArgument3=0  MeasurementFcn4=myMeasurementFcn  HasMeasurementEnablePort4=off  HasAdditiveMeasurementNoise4=Additive  MeasurementNoise4=1  HasTimeVaryingMeasurementNoise4=off  HasMeasurementFcnExtraArgument4=0  MeasurementFcn5=myMeasurementFcn  HasMeasurementEnablePort5=off  HasAdditiveMeasurementNoise5=Additive  MeasurementNoise5=1  HasTimeVaryingMeasurementNoise5=off  HasMeasurementFcnExtraArgument5=0  EnableMultirate=off  StateTransitionFcnSampleTime=1  MeasurementFcn1SampleTime=1  MeasurementFcn2SampleTime=1  MeasurementFcn3SampleTime=1  MeasurementFcn4SampleTime=1  MeasurementFcn5SampleTime=1  UseCurrentEstimator=on  OutputStateCovariance=on  DataType=double  SampleTime=octomodel.sampletime  NumberOfMeasurements=1
      settings: SourceProductBaseCode=CT,DR,TF,ID,NV,AR,RO,VE
  Zero-Order Hold1 : ZeroOrderHold  SampleTime=octomodel.sampletime
  Zero-Order Hold2 : ZeroOrderHold  SampleTime=octomodel.sampletime
  thrust constant : Gain  Gain=octomodel.ct
  ESC Voltage : Outport  VectorParamsAs1DForOutWhenUnconnected=off
  RPM : Outport  Port=2  VectorParamsAs1DForOutWhenUnconnected=off
  ESC Current : Outport  Port=3  VectorParamsAs1DForOutWhenUnconnected=off
  tag scope: motor4=global
  wires:
  Square/1 -> thrust constant/1
  thrust constant/1 -> Terminator/1
  Convert rad/s to rmp/1 -> RPM/1
  StaticTfric/1 -> Mechanical part/1(Static Friction Torque)
  Electrical part/1(Electrical Torque) -> Mechanical part/2(Electrical Torque)
  Mechanical part/2(Torque) -> Terminator1/1
  Control  Voltage/1 -> MATLAB Function1/1(mu), Electrical part/1(ESC voltage), ESC Voltage/1
  Zero-Order Hold1/1 -> Median Filter1/1
  Mechanical part/1(w angular speed) -> Median Filter2/1, Convert rad/s to rmp/1, Square/1, Electrical part/2(w angular speed)
  Electrical part/2(current) -> MATLAB Function/1(mu), ESC Current/1
  MATLAB Function/1(y) -> Zero-Order Hold1/1
  Constant2/1 -> MATLAB Function/2(sigma)
  Constant1/1 -> MATLAB Function1/2(sigma)
  MATLAB Function1/1(y) -> Zero-Order Hold2/1
  Median Filter2/1 -> Rate Transition1/1
  Median Filter1/1 -> Mux/2
  Mux/1 -> Simulink Function/1(Input)
  Rate Transition1/1 -> Mux/1
  Unscented Kalman Filter/1 -> [motor4]
  Constant6/1 -> Simulink Function/2(Input1)
  Zero-Order Hold2/1 -> Unscented Kalman Filter/1, Median Filter/1
  Unscented Kalman Filter/2 -> Terminator2/1

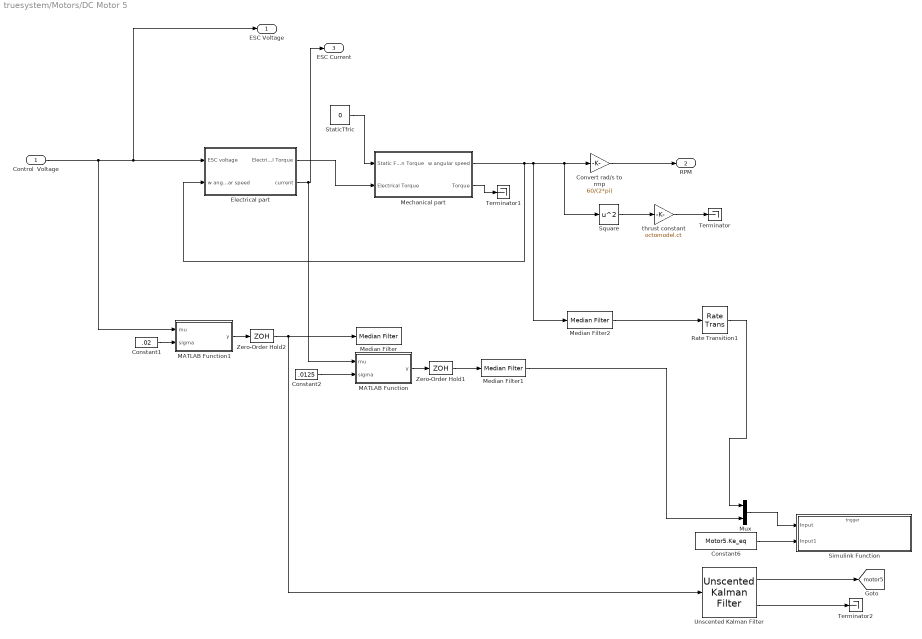
== system truesystem/Motors/DC Motor 5 ==
  Control  Voltage : Inport
  Constant1 : Constant  Value=.02
  Constant2 : Constant  Value=.0125
  Constant6 : Constant  Value=Motor5.Ke_eq
  Convert rad/s to rmp : Gain  Gain=60/(2*pi)
  Electrical part : Subsystem
  MATLAB Function : MATLAB Function  TreatAsAtomicUnit=on
  MATLAB Function1 : MATLAB Function  TreatAsAtomicUnit=on
  Mechanical part : Subsystem
  Median Filter : dspstat3/Median Filter  WindowLength=5  SimulateUsing=Interpreted execution
      settings: SourceProductBaseCode=DS
  Median Filter1 : dspstat3/Median Filter  WindowLength=5  SimulateUsing=Interpreted execution
      settings: SourceProductBaseCode=DS
  Median Filter2 : dspstat3/Median Filter  WindowLength=5  SimulateUsing=Interpreted execution
      settings: SourceProductBaseCode=DS
  Mux : Mux  Inputs=2
  Rate Transition1 : RateTransition  OutPortSampleTime=octomodel.sampletime
  Simulink Function : Subsystem  TreatAsAtomicUnit=on
  Square : Math  Operator=square  SaturateOnIntegerOverflow=on
  StaticTfric : Constant  Value=0
  Terminator : Terminator
  Terminator1 : Terminator
  Terminator2 : Terminator
  Unscented Kalman Filter : sharedTrackingLibrary/Unscented Kalman Filter  StateTransitionFcn=MotorTransitionFcn  HasAdditiveProcessNoise=Additive  ProcessNoise=0.001  HasTimeVaryingProcessNoise=off  HasStateTransitionFcnExtraArgument=0  InitialState=MotorEstimator.Rinit  InitialStateCovariance=0.001  Alpha=0.0001  Beta=2  Kappa=0  MeasurementFcn1=MotorMeasurementFcn5  HasMeasurementEnablePort1=off  HasAdditiveMeasurementNoise1=Additive  MeasurementNoise1=0.02  HasTimeVaryingMeasurementNoise1=off  HasMeasurementFcnExtraArgument1=0  MeasurementFcn2=myMeasurementFcn  HasMeasurementEnablePort2=off  HasAdditiveMeasurementNoise2=Additive  MeasurementNoise2=1  HasTimeVaryingMeasurementNoise2=off  HasMeasurementFcnExtraArgument2=0  MeasurementFcn3=myMeasurementFcn  HasMeasurementEnablePort3=off  HasAdditiveMeasurementNoise3=Additive  MeasurementNoise3=1  HasTimeVaryingMeasurementNoise3=off  HasMeasurementFcnExtraArgument3=0  MeasurementFcn4=myMeasurementFcn  HasMeasurementEnablePort4=off  HasAdditiveMeasurementNoise4=Additive  MeasurementNoise4=1  HasTimeVaryingMeasurementNoise4=off  HasMeasurementFcnExtraArgument4=0  MeasurementFcn5=myMeasurementFcn  HasMeasurementEnablePort5=off  HasAdditiveMeasurementNoise5=Additive  MeasurementNoise5=1  HasTimeVaryingMeasurementNoise5=off  HasMeasurementFcnExtraArgument5=0  EnableMultirate=off  StateTransitionFcnSampleTime=1  MeasurementFcn1SampleTime=1  MeasurementFcn2SampleTime=1  MeasurementFcn3SampleTime=1  MeasurementFcn4SampleTime=1  MeasurementFcn5SampleTime=1  UseCurrentEstimator=on  OutputStateCovariance=on  DataType=double  SampleTime=octomodel.sampletime  NumberOfMeasurements=1
      settings: SourceProductBaseCode=CT,DR,TF,ID,NV,AR,RO,VE
  Zero-Order Hold1 : ZeroOrderHold  SampleTime=octomodel.sampletime
  Zero-Order Hold2 : ZeroOrderHold  SampleTime=octomodel.sampletime
  thrust constant : Gain  Gain=octomodel.ct
  ESC Voltage : Outport  VectorParamsAs1DForOutWhenUnconnected=off
  RPM : Outport  Port=2  VectorParamsAs1DForOutWhenUnconnected=off
  ESC Current : Outport  Port=3  VectorParamsAs1DForOutWhenUnconnected=off
  tag scope: motor5=global
  wires:
  Square/1 -> thrust constant/1
  thrust constant/1 -> Terminator/1
  Convert rad/s to rmp/1 -> RPM/1
  StaticTfric/1 -> Mechanical part/1(Static Friction Torque)
  Electrical part/1(Electrical Torque) -> Mechanical part/2(Electrical Torque)
  Mechanical part/2(Torque) -> Terminator1/1
  Control  Voltage/1 -> MATLAB Function1/1(mu), Electrical part/1(ESC voltage), ESC Voltage/1
  Zero-Order Hold1/1 -> Median Filter1/1
  Mechanical part/1(w angular speed) -> Median Filter2/1, Convert rad/s to rmp/1, Square/1, Electrical part/2(w angular speed)
  Electrical part/2(current) -> MATLAB Function/1(mu), ESC Current/1
  MATLAB Function/1(y) -> Zero-Order Hold1/1
  Constant2/1 -> MATLAB Function/2(sigma)
  Constant1/1 -> MATLAB Function1/2(sigma)
  MATLAB Function1/1(y) -> Zero-Order Hold2/1
  Median Filter2/1 -> Rate Transition1/1
  Median Filter1/1 -> Mux/2
  Mux/1 -> Simulink Function/1(Input)
  Rate Transition1/1 -> Mux/1
  Unscented Kalman Filter/1 -> [motor5]
  Constant6/1 -> Simulink Function/2(Input1)
  Zero-Order Hold2/1 -> Unscented Kalman Filter/1, Median Filter/1
  Unscented Kalman Filter/2 -> Terminator2/1

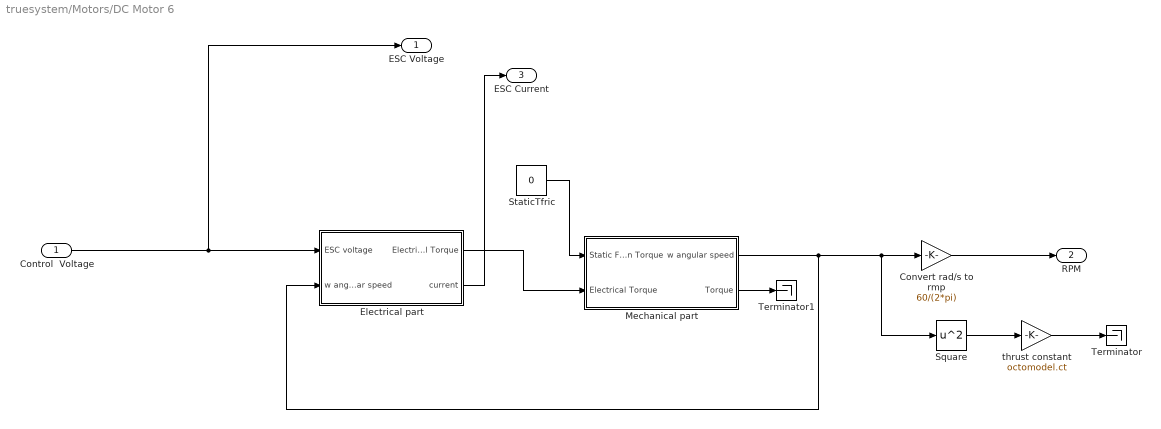
== system truesystem/Motors/DC Motor 6 ==
  Control  Voltage : Inport
  Convert rad/s to rmp : Gain  Gain=60/(2*pi)
  Electrical part : Subsystem
  Mechanical part : Subsystem
  Square : Math  Operator=square  SaturateOnIntegerOverflow=on
  StaticTfric : Constant  Value=0
  Terminator : Terminator
  Terminator1 : Terminator
  thrust constant : Gain  Gain=octomodel.ct
  ESC Voltage : Outport  VectorParamsAs1DForOutWhenUnconnected=off
  RPM : Outport  Port=2  VectorParamsAs1DForOutWhenUnconnected=off
  ESC Current : Outport  Port=3  VectorParamsAs1DForOutWhenUnconnected=off
  wires:
  Square/1 -> thrust constant/1
  Mechanical part/1(w angular speed) -> Convert rad/s to rmp/1, Square/1, Electrical part/2(w angular speed)
  Convert rad/s to rmp/1 -> RPM/1
  Electrical part/2(current) -> ESC Current/1
  Control  Voltage/1 -> Electrical part/1(ESC voltage), ESC Voltage/1
  StaticTfric/1 -> Mechanical part/1(Static Friction Torque)
  Electrical part/1(Electrical Torque) -> Mechanical part/2(Electrical Torque)
  thrust constant/1 -> Terminator/1
  Mechanical part/2(Torque) -> Terminator1/1

== system truesystem/Motors/DC Motor 7 ==
  Control  Voltage : Inport
  Convert rad/s to rmp : Gain  Gain=60/(2*pi)
  Electrical part : Subsystem
  Mechanical part : Subsystem
  Square : Math  Operator=square  SaturateOnIntegerOverflow=on
  StaticTfric : Constant  Value=0
  Terminator : Terminator
  Terminator1 : Terminator
  thrust constant : Gain  Gain=octomodel.ct
  ESC Voltage : Outport  VectorParamsAs1DForOutWhenUnconnected=off
  RPM : Outport  Port=2  VectorParamsAs1DForOutWhenUnconnected=off
  ESC Current : Outport  Port=3  VectorParamsAs1DForOutWhenUnconnected=off
  wires:
  Electrical part/1(Electrical Torque) -> Mechanical part/2(Electrical Torque)
  StaticTfric/1 -> Mechanical part/1(Static Friction Torque)
  Control  Voltage/1 -> ESC Voltage/1, Electrical part/1(ESC voltage)
  Electrical part/2(current) -> ESC Current/1
  Convert rad/s to rmp/1 -> RPM/1
  Mechanical part/1(w angular speed) -> Electrical part/2(w angular speed), Square/1, Convert rad/s to rmp/1
  Square/1 -> thrust constant/1
  thrust constant/1 -> Terminator/1
  Mechanical part/2(Torque) -> Terminator1/1

== system truesystem/Motors/DC Motor 8 ==
  Control  Voltage : Inport
  Convert rad/s to rmp : Gain  Gain=60/(2*pi)
  Electrical part : Subsystem
  Mechanical part : Subsystem
  Square : Math  Operator=square  SaturateOnIntegerOverflow=on
  StaticTfric : Constant  Value=0
  Terminator : Terminator
  Terminator1 : Terminator
  thrust constant : Gain  Gain=octomodel.ct
  ESC Voltage : Outport  VectorParamsAs1DForOutWhenUnconnected=off
  RPM : Outport  Port=2  VectorParamsAs1DForOutWhenUnconnected=off
  ESC Current : Outport  Port=3  VectorParamsAs1DForOutWhenUnconnected=off
  wires:
  Square/1 -> thrust constant/1
  Mechanical part/1(w angular speed) -> Convert rad/s to rmp/1, Square/1, Electrical part/2(w angular speed)
  Convert rad/s to rmp/1 -> RPM/1
  Electrical part/2(current) -> ESC Current/1
  Control  Voltage/1 -> Electrical part/1(ESC voltage), ESC Voltage/1
  StaticTfric/1 -> Mechanical part/1(Static Friction Torque)
  Electrical part/1(Electrical Torque) -> Mechanical part/2(Electrical Torque)
  thrust constant/1 -> Terminator/1
  Mechanical part/2(Torque) -> Terminator1/1

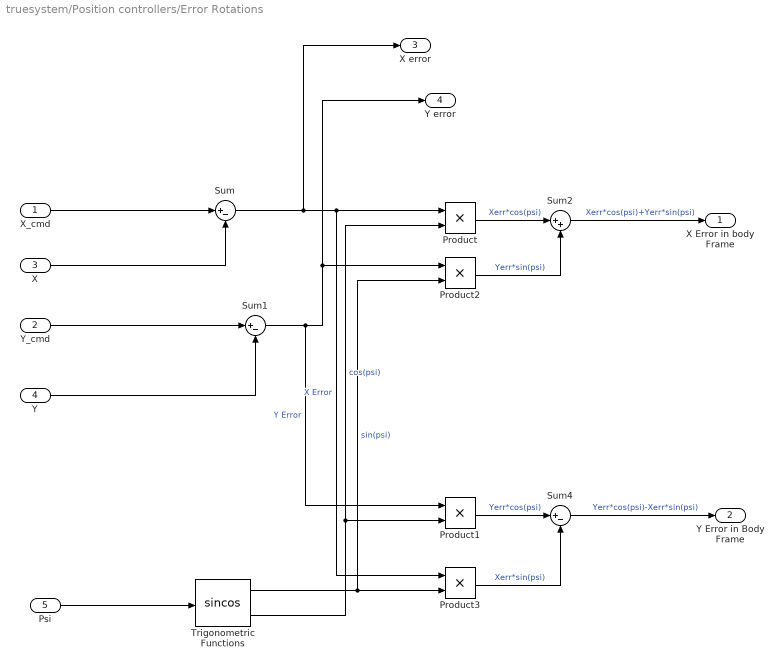
== system truesystem/Position controllers/Error Rotations ==
  X_cmd : Inport
  Y_cmd : Inport  Port=2
  X : Inport  Port=3
  Y : Inport  Port=4
  Psi : Inport  Port=5
  Product{,1..3} (4 alike) : Product
  Sum : Sum  Inputs=|+-
  Sum1 : Sum  Inputs=|+-
  Sum2 : Sum  Inputs=|++
  Sum4 : Sum  Inputs=|+-
  Trigonometric Functions : Trigonometry  Operator=sincos
  X Error in body Frame : Outport  VectorParamsAs1DForOutWhenUnconnected=off
  Y Error in Body Frame : Outport  Port=2  VectorParamsAs1DForOutWhenUnconnected=off
  X error : Outport  Port=3  VectorParamsAs1DForOutWhenUnconnected=off
  "Y error " : Outport  Port=4  VectorParamsAs1DForOutWhenUnconnected=off
  wires:
  Sum4/1 -> Y Error in Body Frame/1  "Yerr*cos(psi)-Xerr*sin(psi)"
  Product3/1 -> Sum4/2  "Xerr*sin(psi)"
  Sum1/1 -> "Y error "/1, Product2/1, Product1/1  "Y Error"
  Trigonometric Functions/1 -> Product2/2, Product3/2  "sin(psi)"
  Sum2/1 -> X Error in body Frame/1  "Xerr*cos(psi)+Yerr*sin(psi)"
  Y_cmd/1 -> Sum1/1
  X_cmd/1 -> Sum/1
  X/1 -> Sum/2
  Y/1 -> Sum1/2
  Sum/1 -> X error/1, Product3/1, Product/1  "X Error"
  Trigonometric Functions/2 -> Product/2, Product1/2  "cos(psi)"
  Product/1 -> Sum2/1  "Xerr*cos(psi)"
  Product2/1 -> Sum2/2  "Yerr*sin(psi)"
  Product1/1 -> Sum4/1  "Yerr*cos(psi)"
  Psi/1 -> Trigonometric Functions/1

== system truesystem/Position controllers/PD_Phi_des ==
  Ydot_ref : Inport
  Ydot : Inport  Port=2
  Add : Sum  Inputs=+-
  Gain : Gain  Gain=0.1
  Gain1 : Gain  Gain=0
  Gain2 : Gain  Gain=-1
  Saturation in radians : Saturate  UpperLimit=12*pi/180  LowerLimit=-12*pi/180
  Sum : Sum  Inputs=|+-
  Phi_des : Outport  VectorParamsAs1DForOutWhenUnconnected=off
  wires:
  Saturation in radians/1 -> Phi_des/1
  Ydot_ref/1 -> Add/1
  Ydot/1 -> Add/2, Gain1/1
  Gain1/1 -> Sum/2
  Add/1 -> Gain/1
  Gain/1 -> Sum/1
  Sum/1 -> Gain2/1
  Gain2/1 -> Saturation in radians/1

== system truesystem/Position controllers/PD_Theta_des ==
  Xdot_ref : Inport
  Xdot : Inport  Port=2
  Add : Sum  Inputs=+-
  Gain : Gain  Gain=0.1
  Gain1 : Gain  Gain=0
  Saturation in radians : Saturate  UpperLimit=12*pi/180  LowerLimit=-12*pi/180
  Sum : Sum  Inputs=|+-
  Theta_des : Outport  VectorParamsAs1DForOutWhenUnconnected=off
  wires:
  Sum/1 -> Saturation in radians/1
  Gain/1 -> Sum/1
  Add/1 -> Gain/1
  Gain1/1 -> Sum/2
  Xdot/1 -> Gain1/1, Add/2
  Xdot_ref/1 -> Add/1
  Saturation in radians/1 -> Theta_des/1

== system truesystem/Motors/DC Motor 1 /Electrical part ==
  ESC voltage : Inport
  w angular speed : Inport  Port=2
  1/R : Gain  Gain=1/Motor1.Req
  Ke (Torque constant)1 : Gain  Gain=Motor1.Ke_eq
  Kt (Torque constant) Kt=Ke for an ideal square wave motor : Gain  Gain=Motor1.Ke_eq
  Saturation : Saturate  UpperLimit=11  LowerLimit=0
  Sum : Sum  Inputs=|+-
  Electrical Torque : Outport  VectorParamsAs1DForOutWhenUnconnected=off
  current : Outport  Port=2  VectorParamsAs1DForOutWhenUnconnected=off
  wires:
  1/R/1 -> Saturation/1  "current i"
  Sum/1 -> 1/R/1
  Kt (Torque constant) Kt=Ke for an ideal square wave motor/1 -> Electrical Torque/1
  Ke (Torque constant)1/1 -> Sum/2
  ESC voltage/1 -> Sum/1
  w angular speed/1 -> Ke (Torque constant)1/1
  Saturation/1 -> Kt (Torque constant) Kt=Ke for an ideal square wave motor/1, current/1

== system truesystem/Motors/DC Motor 1 /Mechanical part ==
  Static Friction Torque : Inport
  Electrical Torque : Inport  Port=2
  1/J Inertia constant : Gain  Gain=1/Motor1.J
  "Df viscous damping coefficient Dynamic Friction coefficient " : Gain  Gain=Motor1.Df
  Discrete-Time Integrator : DiscreteIntegrator  gainval=1  InitialCondition=IC.w1  SampleTime=octomodel.sampletime  ICPrevOutput=DiscIntNeverNeededParam  ICPrevScaledInput=DiscIntNeverNeededParam
  Gain : Gain  Gain=Motor1.cq
  Square : Math  Operator=square  SaturateOnIntegerOverflow=on
  Sum1 : Sum  Inputs=--+-
  w angular speed : Outport  VectorParamsAs1DForOutWhenUnconnected=off
  Torque : Outport  Port=2  VectorParamsAs1DForOutWhenUnconnected=off
  wires:
  1/J Inertia constant/1 -> Discrete-Time Integrator/1
  Static Friction Torque/1 -> Sum1/2
  "Df viscous damping coefficient Dynamic Friction coefficient "/1 -> Sum1/4
  Discrete-Time Integrator/1 -> w angular speed/1, Square/1, "Df viscous damping coefficient Dynamic Friction coefficient "/1  "w angular speed"
  Sum1/1 -> 1/J Inertia constant/1
  Electrical Torque/1 -> Sum1/3
  Gain/1 -> Torque/1, Sum1/1
  Square/1 -> Gain/1

== system truesystem/Motors/DC Motor 2/Electrical part ==
  ESC voltage : Inport
  w angular speed : Inport  Port=2
  1/R : Gain  Gain=1/Motor2.Req
  Ke (Torque constant)1 : Gain  Gain=Motor2.Ke_eq
  Kt (Torque constant) Kt=Ke for an ideal square wave motor : Gain  Gain=Motor2.Ke_eq
  Saturation : Saturate  UpperLimit=11  LowerLimit=0
  Scope1 : Scope
  Scope2 : Scope
  Scope3 : Scope
  Sum : Sum  Inputs=|+-
  Electrical Torque : Outport  VectorParamsAs1DForOutWhenUnconnected=off
  current : Outport  Port=2  VectorParamsAs1DForOutWhenUnconnected=off
  wires:
  Saturation/1 -> current/1, Kt (Torque constant) Kt=Ke for an ideal square wave motor/1, Scope1/1
  w angular speed/1 -> Ke (Torque constant)1/1
  ESC voltage/1 -> Sum/1
  Ke (Torque constant)1/1 -> Sum/2, Scope2/1
  Kt (Torque constant) Kt=Ke for an ideal square wave motor/1 -> Electrical Torque/1
  Sum/1 -> 1/R/1, Scope3/1
  1/R/1 -> Saturation/1  "current i"

== system truesystem/Motors/DC Motor 2/Mechanical part ==
  Static Friction Torque : Inport
  Electrical Torque : Inport  Port=2
  1/J Inertia constant : Gain  Gain=1/Motor2.J
  "Df viscous damping coefficient Dynamic Friction coefficient " : Gain  Gain=Motor2.Df
  Discrete-Time Integrator : DiscreteIntegrator  gainval=1  InitialCondition=IC.w2  SampleTime=octomodel.sampletime  ICPrevOutput=DiscIntNeverNeededParam  ICPrevScaledInput=DiscIntNeverNeededParam
  Gain : Gain  Gain=Motor2.cq
  Square : Math  Operator=square  SaturateOnIntegerOverflow=on
  Sum1 : Sum  Inputs=--+-
  w angular speed : Outport  VectorParamsAs1DForOutWhenUnconnected=off
  Torque : Outport  Port=2  VectorParamsAs1DForOutWhenUnconnected=off
  wires:
  Square/1 -> Gain/1
  Gain/1 -> Sum1/1, Torque/1
  Electrical Torque/1 -> Sum1/3
  Sum1/1 -> 1/J Inertia constant/1
  Discrete-Time Integrator/1 -> "Df viscous damping coefficient Dynamic Friction coefficient "/1, Square/1, w angular speed/1  "w angular speed"
  "Df viscous damping coefficient Dynamic Friction coefficient "/1 -> Sum1/4
  Static Friction Torque/1 -> Sum1/2
  1/J Inertia constant/1 -> Discrete-Time Integrator/1

== system truesystem/Motors/DC Motor 2/Simulink Function ==
  Input : Inport  PortDimensions=2
  Input1 : Inport  Port=2
  MotorMeasurementFcn2 : TriggerPort  TriggerType=function-call  IsSimulinkFunction=on  FunctionName=MotorMeasurementFcn2  VariantControl=(inherit)
  MATLAB Function : MATLAB Function  TreatAsAtomicUnit=on
  x : ArgIn  DisableCoverage=on  ArgumentName=x
  xNext : ArgOut  DisableCoverage=on  ArgumentName=xNext
  wires:
  x/1 -> MATLAB Function/1("x ")
  MATLAB Function/1(x) -> xNext/1
  Input/1 -> MATLAB Function/2(u)
  Input1/1 -> MATLAB Function/3(param)

== system truesystem/Motors/DC Motor 3/Electrical part ==
  ESC voltage : Inport
  w angular speed : Inport  Port=2
  1/R : Gain  Gain=1/Motor3.Req
  Ke (Torque constant)1 : Gain  Gain=Motor3.Ke_eq
  Kt (Torque constant) Kt=Ke for an ideal square wave motor : Gain  Gain=Motor3.Ke_eq
  Saturation : Saturate  UpperLimit=11  LowerLimit=0
  Sum : Sum  Inputs=|+-
  Electrical Torque : Outport  VectorParamsAs1DForOutWhenUnconnected=off
  current : Outport  Port=2  VectorParamsAs1DForOutWhenUnconnected=off
  wires:
  1/R/1 -> Saturation/1  "current i"
  Sum/1 -> 1/R/1
  Kt (Torque constant) Kt=Ke for an ideal square wave motor/1 -> Electrical Torque/1
  Ke (Torque constant)1/1 -> Sum/2
  ESC voltage/1 -> Sum/1
  w angular speed/1 -> Ke (Torque constant)1/1
  Saturation/1 -> Kt (Torque constant) Kt=Ke for an ideal square wave motor/1, current/1
